simulink model "Frequecy_Analysis"  (R2016a)
settings: Solver=VariableStepAuto  StartTime=0.0  StopTime=10  RelTol=1e-3
libraries: simulink x2
settings Model: Creator=73565  LastModifiedBy=Administrator

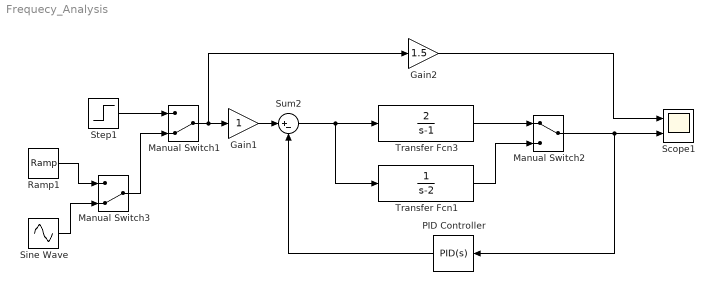
== system Frequecy_Analysis ==
  Gain1 : Gain
  Gain2 : Gain  Gain=1.5
  Manual Switch1 : ManualSwitch  CurrentSetting=0
  Manual Switch2 : ManualSwitch
  Manual Switch3 : ManualSwitch  CurrentSetting=0
  PID Controller : simulink/Continuous/PID Controller  Controller=PID  TimeDomain=Continuous-time  SampleTime=-1  IntegratorMethod=Forward Euler  FilterMethod=Forward Euler  Form=Parallel  UseFilter=on  ControllerParametersSource=internal  P=1  I=0  D=0  N=100  InitialConditionSource=internal  InitialConditionForIntegrator=0  InitialConditionForFilter=0  ExternalReset=none  LimitOutput=off  UpperSaturationLimit=inf  LowerSaturationLimit=-inf  LinearizeAsGain=on  AntiWindupMode=none  Kb=1  TrackingMode=off  Kt=1  PParamMin=[]  PParamMax=[]  IParamMin=[]  IParamMax=[]  DParamMin=[]  DParamMax=[]  NParamMin=[]  NParamMax=[]  KbParamMin=[]  KbParamMax=[]  KtParamMin=[]  KtParamMax=[]  POutMin=[]  POutMax=[]  IOutMin=[]  IOutMax=[]  DOutMin=[]  DOutMax=[]  NOutMin=[]  NOutMax=[]  KbOutMin=[]  KbOutMax=[]  KtOutMin=[]  KtOutMax=[]  IntegratorOutMin=[]  IntegratorOutMax=[]  FilterOutMin=[]  FilterOutMax=[]  SumOutMin=[]  SumOutMax=[]  SumI1OutMin=[]  SumI1OutMax=[]  SumI2OutMin=[]  SumI2OutMax=[]  SumI3OutMin=[]  SumI3OutMax=[]  SumDOutMin=[]  SumDOutMax=[]  SaturationOutMin=[]  SaturationOutMax=[]  IntegratorContinuousStateAttributes=''  IntegratorStateMustResolveToSignalObject=off  IntegratorRTWStateStorageClass=Auto  FilterContinuousStateAttributes=''  FilterStateMustResolveToSignalObject=off  FilterRTWStateStorageClass=Auto  DifferentiatorICPrevScaledInput=0  DifferentiatorOutMin=[]  DifferentiatorOutMax=[]
  Ramp1 : simulink/Sources/Ramp  slope=1  start=0  X0=0
  Scope1 : Scope  NumInputPorts=2
  Sine Wave : Sin  Phase=0*pi/9  SampleTime=0
  Step1 : Step  SampleTime=0
  Sum2 : Sum  Inputs=|+-
  Transfer Fcn1 : TransferFcn  Denominator=[1 -2]
  Transfer Fcn3 : TransferFcn  Numerator=[2]  Denominator=[1 -1]
  wires:
  Step1/1 -> Manual Switch1/1
  PID Controller/1 -> Sum2/2
  Transfer Fcn3/1 -> Manual Switch2/1
  Manual Switch2/1 -> Scope1/2, PID Controller/1
  Sum2/1 -> Transfer Fcn1/1, Transfer Fcn3/1
  Manual Switch1/1 -> Gain2/1, Gain1/1
  Gain1/1 -> Sum2/1
  Manual Switch3/1 -> Manual Switch1/2
  Ramp1/1 -> Manual Switch3/1
  Sine Wave/1 -> Manual Switch3/2
  Gain2/1 -> Scope1/1
  Transfer Fcn1/1 -> Manual Switch2/2
